simulink model "clab3_1_sim"  (R2014a)
settings: Solver=ode45  StartTime=0.0  StopTime=10.0  RelTol=1e-3
values from neighbouring files (symbols this model uses):
  alpha = 7600    [clab3_1.m]    (also in clab3_2.m)
  beta = 2000    [clab3_1.m]    (also in clab3_2.m = 1430)
  lamda = 2470    [clab3_1.m]
  mu = 7200    [clab3_1.m]    (also in clab3_2.m)
  phi = 0.51    [clab3_1.m]    (also in clab3_2.m)
  Ql = 8400    [clab3_1.m]    (also in clab3_2.m)
  theta = 2.5    [clab3_1.m]    (also in clab3_2.m)
  v = 139000    [clab3_1.m]    (also in clab3_2.m = 70000)
settings Model: Creator=Tommy  LastModifiedBy=Tommy

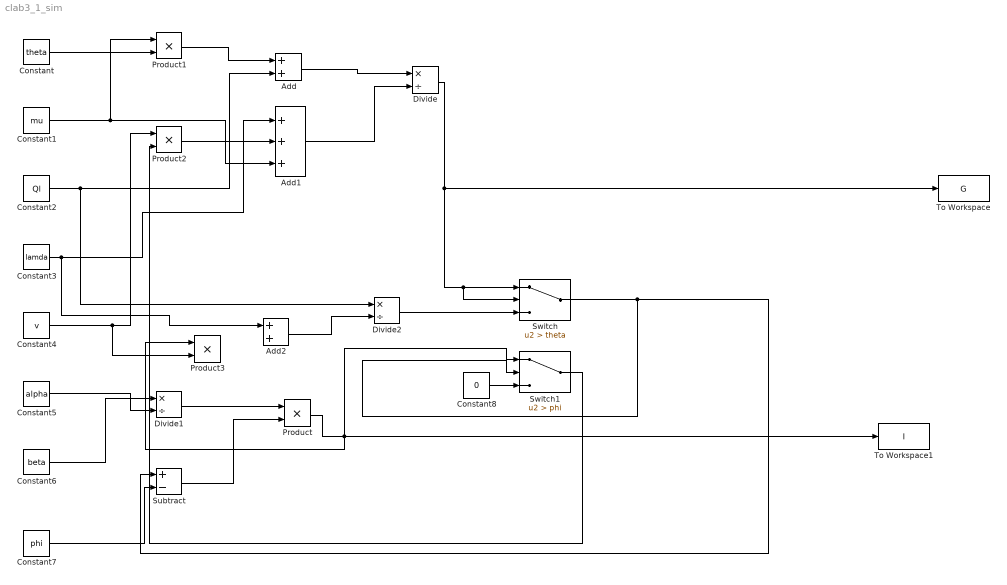
== system clab3_1_sim ==
  Add : Sum
  Add1 : Sum  Inputs=+++
  Add2 : Sum
  Constant : Constant  Value=theta
  Constant1 : Constant  Value=mu
  Constant2 : Constant  Value=Ql
  Constant3 : Constant  Value=lamda
  Constant4 : Constant  Value=v
  Constant5 : Constant  Value=alpha
  Constant6 : Constant  Value=beta
  Constant7 : Constant  Value=phi
  Constant8 : Constant  Value=0
  Divide : Product  Inputs=*/
  Divide1 : Product  Inputs=*/
  Divide2 : Product  Inputs=*/
  Product{,1..3} (4 alike) : Product
  Subtract : Sum  Inputs=+-
  Switch : Switch  Criteria=u2 > Threshold  Threshold=theta
  Switch1 : Switch  Criteria=u2 > Threshold  Threshold=phi
  To Workspace : ToWorkspace  VariableName=G  SaveFormat=Timeseries  SampleTime=-1
  To Workspace1 : ToWorkspace  VariableName=I  SaveFormat=Timeseries  SampleTime=-1
  wires:
  Constant3/1 -> Add2/1, Add1/1
  Constant1/1 -> Add1/3, Product1/1
  Product1/1 -> Add/1
  Constant2/1 -> Divide2/1, Add/2
  Add/1 -> Divide/1
  Constant4/1 -> Product3/2, Product2/1
  Product2/1 -> Add1/2
  Constant/1 -> Product1/2
  Add1/1 -> Divide/2
  Constant6/1 -> Divide1/1
  Constant5/1 -> Divide1/2
  Divide1/1 -> Product/1
  Divide/1 -> Switch/2, Switch/1, To Workspace/1
  Constant7/1 -> Subtract/2
  Subtract/1 -> Product/2
  Product/1 -> Product3/1, Switch1/1, To Workspace1/1
  Switch/1 -> Switch1/2, Subtract/1
  Constant8/1 -> Switch1/3
  Add2/1 -> Divide2/2
  Divide2/1 -> Switch/3
  Switch1/1 -> Product2/2
